simulink model "mySimulinkModel"  (R2025b)
settings: Solver=FixedStepAuto  StartTime=0.0  StopTime=50  RelTol=1e-3
settings Model: Creator=samar  LastModifiedBy=dsamarka

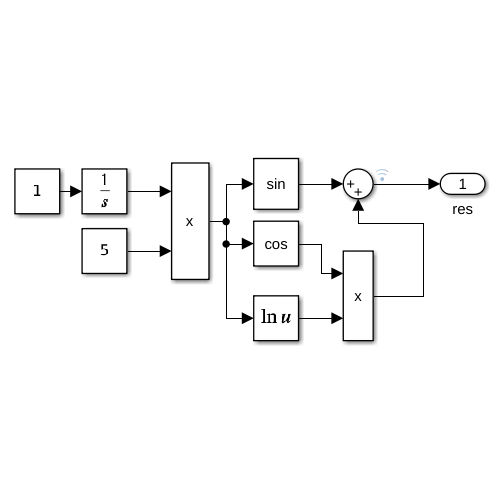
[thumbnail: Simulink's stored preview of the top-level diagram]
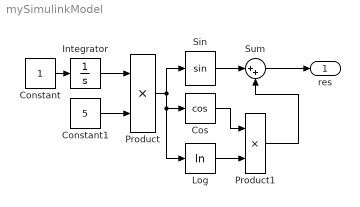
== system mySimulinkModel ==
  Constant : Constant
  Constant1 : Constant  Value=5
  Cos : Trigonometry  Operator=cos
  Integrator : Integrator
  Log : Math  Operator=log
  Product : Product
  Product1 : Product
  Sin : Trigonometry
  Sum : Sum  Inputs=|++
  res : Outport
  wires:
  Constant/1 -> Integrator/1
  Integrator/1 -> Product/1
  Constant1/1 -> Product/2
  Product/1 -> Log/1, Cos/1, Sin/1
  Sin/1 -> Sum/1
  Sum/1 -> res/1
  Log/1 -> Product1/2
  Cos/1 -> Product1/1
  Product1/1 -> Sum/2
